simulink model "i_regulator"  (R2026a)
settings: Solver=VariableStepAuto  StopTime=12000
values from neighbouring files (symbols this model uses):
  K_I = 0.0005    [lab3.m]
  K_mech = 1    [lab3.m]    (also in lab3_auto.m)
  K_obj = 1    [lab3.m]    (also in lab3_auto.m)
  K_sens = 3.9    [lab3.m]    (also in lab3_auto.m)
  T1 = 100    [lab3.m]    (also in lab3_auto.m)
  T2 = 250    [lab3.m]    (also in lab3_auto.m)
  T_sens = 20    [lab3.m]    (also in lab3_auto.m)
libraries: sdolib x1
settings Model: Creator=Lenovo  LastModifiedBy=Lenovo

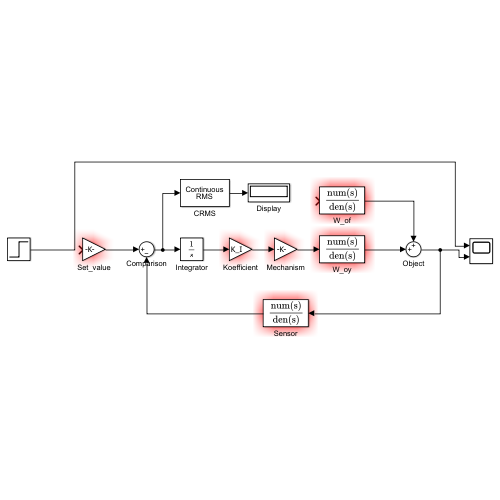
[thumbnail: Simulink's stored preview of the top-level diagram]
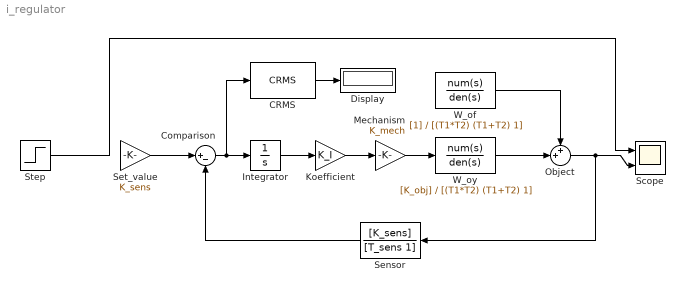
== system i_regulator ==
  CRMS : sdolib/RMS Blocks/CRMS
  Comparison : Sum  Inputs=|+-
  Display : Display
  Integrator : Integrator
  Koefficient : Gain  Gain=K_I
  Mechanism : Gain  Gain=K_mech
  Object : Sum  Inputs=++|
  Scope : Scope  NumInputPorts=2
      settings: ActiveDisplayYMinimum=-0.12611547419634386  ActiveDisplayYMaximum=1.1350392677670951
  Sensor : TransferFcn  Numerator=[K_sens]  Denominator=[T_sens 1]
  Set_value : Gain  Gain=K_sens
  Step : Step  Time=0  SampleTime=0
  W_of : TransferFcn  Denominator=[(T1*T2) (T1+T2) 1]
  W_oy : TransferFcn  Numerator=[K_obj]  Denominator=[(T1*T2) (T1+T2) 1]
  wires:
  W_of/1 -> Object/1
  Mechanism/1 -> W_oy/1
  Koefficient/1 -> Mechanism/1
  Set_value/1 -> Comparison/1
  Sensor/1 -> Comparison/2
  Step/1 -> Scope/1
  W_oy/1 -> Object/2
  Object/1 -> Sensor/1, Scope/2
  Comparison/1 -> CRMS/1, Integrator/1
  Integrator/1 -> Koefficient/1
  CRMS/1 -> Display/1
